simulink model "baseline64bit"  (R2020b)
settings: Solver=FixedStepDiscrete  StartTime=0.0  StopTime=1  FixedStep=1/1082880  RelTol=1e-3
InitFcn:
  | Ts = 1e-3;
  | Ts_240p = 402*324*Ts;
libraries: hdlsllib x20, visionhdlio x3, visionsources x2
settings Model: DataTypeOverride=Off  ModifiedByFormat=The MathWorks Inc.  Creator=The MathWorks, Inc.  LastModifiedBy=The MathWorks Inc.
settings DataIOCC: LimitDataPoints=on  SaveFormat=Array  SaveOutput=off  SaveTime=off  ReturnWorkspaceOutputs=off
settings OptimizationCC: BlockReduction=off  ConditionallyExecuteInputs=off  DefaultParameterBehavior=Inlined  LifeSpan=inf
settings DebuggingCC: AlgebraicLoopMsg=error  SolverPrmCheckMsg=warning  SingleTaskRateTransMsg=error  ParameterPrecisionLossMsg=none  AllowSymbolicDim=off  SFUnexpectedBacktrackingDiag=warning  SFNoUnconditionalDefaultTransitionDiag=warning  SFExecutionAtInitializationDiag=none  IntegerSaturationMsg=none  ArithmeticOperatorsInVariantConditions=warning
settings HardwareCC: ProdBitPerPointer=32  ProdBitPerSizeT=32  ProdBitPerPtrDiffT=32  ProdLargestAtomicFloat=None  ProdIntDivRoundTo=Undefined  ProdEndianess=Unspecified  ProdWordSize=32  ProdHWDeviceType=ASIC/FPGA->ASIC/FPGA  ProdEqTarget=off
settings ModelReferenceCC: PropagateSignalLabelsOutOfModel=off
settings SFSimCC: SimUseLocalCustomCode=off  CustomCodeUndefinedFunction=UseInterfaceOnly
settings RTWCC: RTWUseLocalCustomCode=off
settings CodeAppCC: StateflowObjectComments=on
settings GRTTargetCC: TargetLangStandard=C89/C90 (ANSI)
settings ConfigComp: CovMetricSettings=dw  CovSaveCumulativeToWorkspaceVar=on  CovSaveSingleToWorkspaceVar=on  CovExternalEMLEnable=off  CovSFcnEnable=off

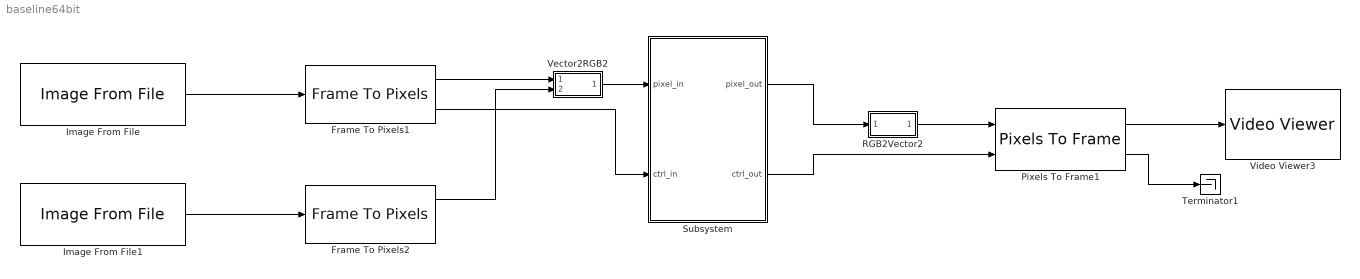
== system baseline64bit ==
  Frame To Pixels1 : visionhdlio/Frame To Pixels  NumComponents=3  NumPixels=1  VideoFormat=Custom  ActivePixelsPerLine=752  ActiveVideoLines=480  TotalPixelsPerLine=752  TotalVideoLines=480  StartingActiveLine=1  FrontPorch=0  SampleTime=0
      settings: SourceProductBaseCode=VT
  Frame To Pixels2 : visionhdlio/Frame To Pixels  NumComponents=3  NumPixels=1  VideoFormat=Custom  ActivePixelsPerLine=752  ActiveVideoLines=480  TotalPixelsPerLine=752  TotalVideoLines=480  StartingActiveLine=1  FrontPorch=0  SampleTime=0
      settings: SourceProductBaseCode=VT
  Image From File : visionsources/Image From File  Tag=vipblks_nd  FileName=left1.bmp  Ts=1  imagePorts=One multidimensional signal  OutPortLabels=R|G|B  ImageDataType=Inherit from input image  sdImageDataType=uint(8)  Signed=on  WordLength=16  FractionLengthMode=User-defined  FractionLength=15
  Image From File1 : visionsources/Image From File  Tag=vipblks_nd  FileName=right1.bmp  Ts=1  imagePorts=One multidimensional signal  OutPortLabels=R|G|B  ImageDataType=Inherit from input image  sdImageDataType=uint(8)  Signed=on  WordLength=16  FractionLengthMode=User-defined  FractionLength=15
  Pixels To Frame1 : visionhdlio/Pixels To Frame  NumComponents=3  NumPixels=1  VideoFormat=Custom  ActivePixelsPerLine=752  ActiveVideoLines=480  TotalPixelsPerLine=752  TotalVideoLines=480
      settings: SourceProductBaseCode=VT
  RGB2Vector2 : Subsystem
  Subsystem : Subsystem  TreatAsAtomicUnit=on
  Terminator1 : Terminator
  Vector2RGB2 : Subsystem
  Video Viewer3 : VideoViewer  FigPos=[1 718 1280 622.666666666667]
  wires:
  Image From File/1 -> Frame To Pixels1/1
  Pixels To Frame1/1 -> Video Viewer3/1
  Pixels To Frame1/2 -> Terminator1/1
  Frame To Pixels1/1 -> Vector2RGB2/1(RGBVector)
  RGB2Vector2/1(RGBVector) -> Pixels To Frame1/1
  Subsystem/1(pixel_out) -> RGB2Vector2/1(RGB)
  Frame To Pixels1/2 -> Subsystem/2(ctrl_in)
  Subsystem/2(ctrl_out) -> Pixels To Frame1/2
  Image From File1/1 -> Frame To Pixels2/1
  Vector2RGB2/1(RGB) -> Subsystem/1(pixel_in)
  Frame To Pixels2/1 -> Vector2RGB2/2(RGBVector1)

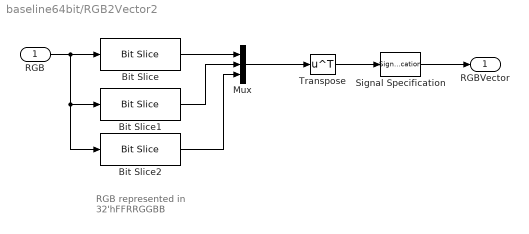
== system baseline64bit/RGB2Vector2 ==
  note: RGB represented in
      | 32'hFFRRGGBB
  RGB : Inport
  Bit Slice : hdlsllib/Logic and Bit Operations/Bit Slice  lidx=23  ridx=16
      settings: SourceProductBaseCode=SL
  Bit Slice1 : hdlsllib/Logic and Bit Operations/Bit Slice  lidx=15  ridx=8
      settings: SourceProductBaseCode=SL
  Bit Slice2 : hdlsllib/Logic and Bit Operations/Bit Slice  lidx=7  ridx=0
      settings: SourceProductBaseCode=SL
  Mux : Mux  Inputs=3
  Signal Specification : SignalSpecification
  Transpose : Math  Operator=transpose  SignedPower=on  SaturateOnIntegerOverflow=on
  RGBVector : Outport  VectorParamsAs1DForOutWhenUnconnected=off
  wires:
  Signal Specification/1 -> RGBVector/1
  Transpose/1 -> Signal Specification/1
  RGB/1 -> Bit Slice/1, Bit Slice1/1, Bit Slice2/1
  Bit Slice1/1 -> Mux/2
  Bit Slice2/1 -> Mux/3
  Bit Slice/1 -> Mux/1
  Mux/1 -> Transpose/1

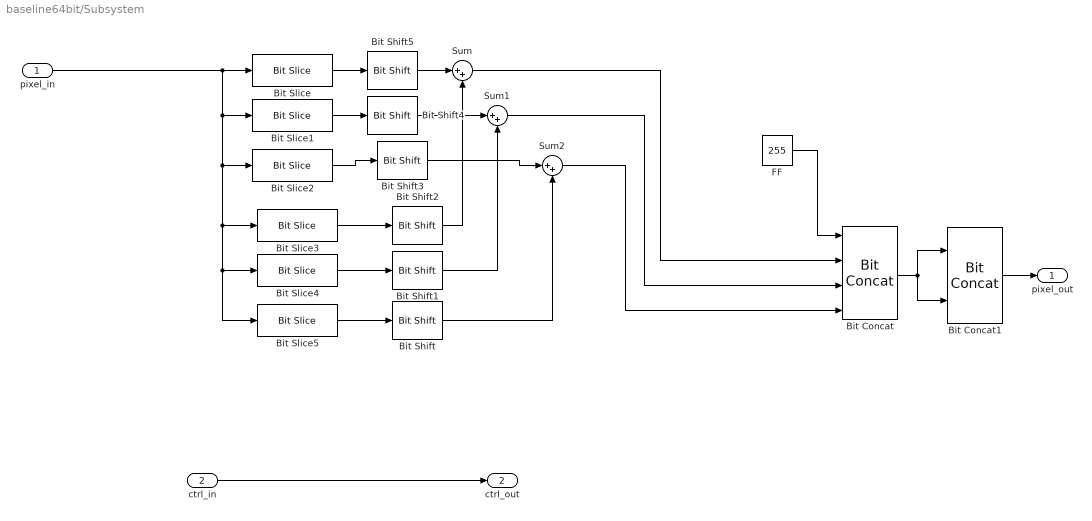
== system baseline64bit/Subsystem ==
  pixel_in : Inport
  ctrl_in : Inport  Port=2
  Bit Concat : hdlsllib/Logic and Bit Operations/Bit Concat  numInputs=4
  Bit Concat1 : hdlsllib/Logic and Bit Operations/Bit Concat  numInputs=2
  Bit Shift{,1..5} (6 alike) : hdlsllib/Logic and Bit Operations/Bit Shift  mode=Shift Right Arithmetic  N=1
  Bit Slice : hdlsllib/Logic and Bit Operations/Bit Slice  lidx=23  ridx=16
      settings: SourceProductBaseCode=SL
  Bit Slice1 : hdlsllib/Logic and Bit Operations/Bit Slice  lidx=15  ridx=8
      settings: SourceProductBaseCode=SL
  Bit Slice2 : hdlsllib/Logic and Bit Operations/Bit Slice  lidx=7  ridx=0
      settings: SourceProductBaseCode=SL
  Bit Slice3 : hdlsllib/Logic and Bit Operations/Bit Slice  lidx=55  ridx=48
      settings: SourceProductBaseCode=SL
  Bit Slice4 : hdlsllib/Logic and Bit Operations/Bit Slice  lidx=47  ridx=40
      settings: SourceProductBaseCode=SL
  Bit Slice5 : hdlsllib/Logic and Bit Operations/Bit Slice  lidx=39  ridx=32
      settings: SourceProductBaseCode=SL
  FF : Constant  Value=255  OutDataTypeStr=uint8  SampleTime=-1
  Sum : Sum  Inputs=|++  OutDataTypeStr=uint8  SaturateOnIntegerOverflow=on
  Sum1 : Sum  Inputs=|++  OutDataTypeStr=uint8  SaturateOnIntegerOverflow=on
  Sum2 : Sum  Inputs=|++  OutDataTypeStr=uint8  SaturateOnIntegerOverflow=on
  pixel_out : Outport  VectorParamsAs1DForOutWhenUnconnected=off
  ctrl_out : Outport  Port=2  VectorParamsAs1DForOutWhenUnconnected=off
  wires:
  ctrl_in/1 -> ctrl_out/1
  Bit Slice/1 -> Bit Shift5/1
  FF/1 -> Bit Concat/1
  Bit Slice2/1 -> Bit Shift3/1
  Bit Slice1/1 -> Bit Shift4/1
  Sum2/1 -> Bit Concat/4
  Sum1/1 -> Bit Concat/3
  Sum/1 -> Bit Concat/2
  Bit Slice3/1 -> Bit Shift2/1
  Bit Slice4/1 -> Bit Shift1/1
  Bit Slice5/1 -> Bit Shift/1
  pixel_in/1 -> Bit Slice/1, Bit Slice1/1, Bit Slice3/1, Bit Slice4/1, Bit Slice5/1, Bit Slice2/1
  Bit Shift/1 -> Sum2/2
  Bit Shift1/1 -> Sum1/2
  Bit Shift2/1 -> Sum/2
  Bit Shift3/1 -> Sum2/1
  Bit Shift4/1 -> Sum1/1
  Bit Shift5/1 -> Sum/1
  Bit Concat1/1 -> pixel_out/1
  Bit Concat/1 -> Bit Concat1/2, Bit Concat1/1

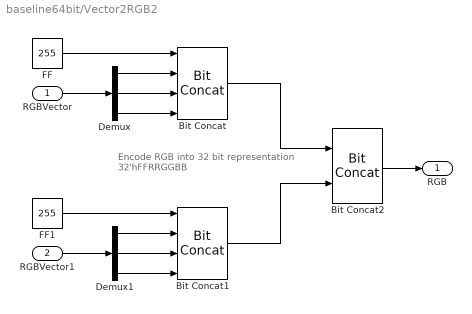
== system baseline64bit/Vector2RGB2 ==
  note: Encode RGB into 32 bit representation
      | 32'hFFRRGGBB
  RGBVector : Inport
  RGBVector1 : Inport  Port=2
  Bit Concat : hdlsllib/Logic and Bit Operations/Bit Concat  numInputs=4
  Bit Concat1 : hdlsllib/Logic and Bit Operations/Bit Concat  numInputs=4
  Bit Concat2 : hdlsllib/Logic and Bit Operations/Bit Concat  numInputs=2
  Demux : Demux  Outputs=3
  Demux1 : Demux  Outputs=3
  FF : Constant  Value=255  OutDataTypeStr=uint8  SampleTime=-1
  FF1 : Constant  Value=255  OutDataTypeStr=uint8  SampleTime=-1
  RGB : Outport  VectorParamsAs1DForOutWhenUnconnected=off
  wires:
  Demux/3 -> Bit Concat/4
  Demux/2 -> Bit Concat/3
  Demux/1 -> Bit Concat/2
  FF/1 -> Bit Concat/1
  RGBVector/1 -> Demux/1
  Demux1/1 -> Bit Concat1/2
  Demux1/2 -> Bit Concat1/3
  Demux1/3 -> Bit Concat1/4
  Bit Concat1/1 -> Bit Concat2/2
  FF1/1 -> Bit Concat1/1
  RGBVector1/1 -> Demux1/1
  Bit Concat2/1 -> RGB/1
  Bit Concat/1 -> Bit Concat2/1
